simulink library "Lib_PFSys_CurrentLimiter_TMATS"  (R2017a)
settings: Solver=ode45  StartTime=0.0  StopTime=10.0  RelTol=1e-3  EnableMultiTasking=on
libraries: Lib_PF_BusLoadDC_TMATS x1
Description:
  | Thomas Modules
settings Model: Creator=jwchapm2  LastModifiedBy=glthoma1
settings DataIOCC: LimitDataPoints=on  SaveFormat=Array
settings OptimizationCC: ExpressionDepthLimit=2147483647  LifeSpan=inf
settings DebuggingCC: UnderspecifiedInitializationDetection=Classic  MergeDetectMultiDrivingBlocksExec=none  SolverPrmCheckMsg=warning  StateNameClashWarn=warning  SFUnexpectedBacktrackingDiag=warning  SFNoUnconditionalDefaultTransitionDiag=warning  SFExecutionAtInitializationDiag=none
settings HardwareCC: ProdBitPerPointer=32  ProdBitPerSizeT=32  ProdBitPerPtrDiffT=32  ProdLargestAtomicFloat=None  ProdIntDivRoundTo=Undefined  ProdEndianess=Unspecified  ProdWordSize=32  ProdHWDeviceType=32-bit Generic
settings ModelReferenceCC: PropagateSignalLabelsOutOfModel=off
settings GRTTargetCC: TargetLangStandard=C89/C90 (ANSI)  GeneratePreprocessorConditionals=Disable all
settings ConfigComp: CovMetricSettings=dw  CovHtmlReporting=on  CovSaveCumulativeToWorkspaceVar=on  CovSaveSingleToWorkspaceVar=on  CovExternalEMLEnable=off

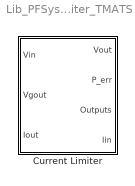
== system Lib_PFSys_CurrentLimiter_TMATS ==
  Current Limiter : Subsystem  mask(Current Limiter){ROn_M=0.01, ROff_M=0.01, IMax_M=1, IMin_M=-1, Rolloff_M=0}
      mask prompts: ROn_M "ROn_M - 'On' Resistance, Ohms"; ROff_M "ROff_M - 'Off' (HiZ) Resistance, Ohms"; IMax_M "IMax_M - Maximum Output Current, Amps"; IMin_M "IMin_M - Minimum Output Current, Amps"; Rolloff_M "Rolloff_M - Rolloff of Impedance Chracteristic as a function of Current (base of exponent)"
      mask help:
      | This block represents a generic current limiting device.
      | If the current through this device is within the upper/lower limits,
      | this device's impedance will be the "On Resistance." Otherwise
      | the impedance will be the "HiZ Resistance."
      |
      | If current is close to the bounds, the impedance will be
      | somewhere in between (the R vs I characteristic is sigmoidal.)
      | You can adjust the rolloff of the characteristic via the rolloff_M
      | parameter, which is the base of the sigmoid function's exponent.

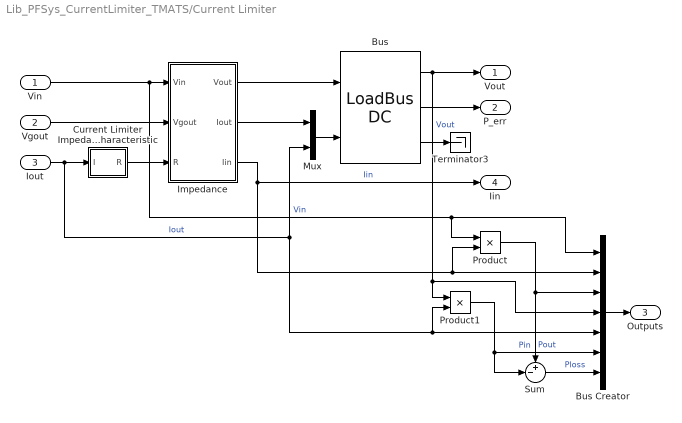
== system Lib_PFSys_CurrentLimiter_TMATS/Current Limiter ==
  Vin : Inport
  Vgout : Inport  Port=2
  Iout : Inport  Port=3
  Bus : Lib_PF_BusLoadDC_TMATS/LoadBus DC  PeInEN_M=off  P_M=0  BlkNm_M=double(gcb)
  Bus Creator : BusCreator  Inputs=7
  Current Limiter Impedance Characteristic : Subsystem
  Impedance : Subsystem
  Mux : Mux  Inputs=2
  Product : Product
  Product1 : Product
  Sum : Sum  Inputs=+-|
  Terminator3 : Terminator
  Vout : Outport
  P_err : Outport  Port=2
  Outputs : Outport  Port=3
  Iin : Outport  Port=4
  wires:
  Iout/1 -> Current Limiter Impedance Characteristic/1(I), Mux/2, Product1/2, Bus Creator/5  "Iout"
  Impedance/2(Iout) -> Mux/1
  Bus/1 -> Product1/1, Bus Creator/4, Vout/1  "Vout"
  Product1/1 -> Bus Creator/6, Sum/2  "Pout"
  Bus Creator/1 -> Outputs/1
  Vin/1 -> Product/1, Bus Creator/1, Impedance/1(Vin)  "Vin"
  Impedance/3(Iin) -> Product/2, Bus Creator/2, Iin/1  "Iin"
  Impedance/1(Vout) -> Bus/1
  Mux/1 -> Bus/2
  Vgout/1 -> Impedance/2(Vgout)
  Sum/1 -> Bus Creator/7  "Ploss"
  Bus/2 -> P_err/1
  Product/1 -> Bus Creator/3, Sum/1  "Pin"
  Bus/3 -> Terminator3/1
  Current Limiter Impedance Characteristic/1(R) -> Impedance/3(R)

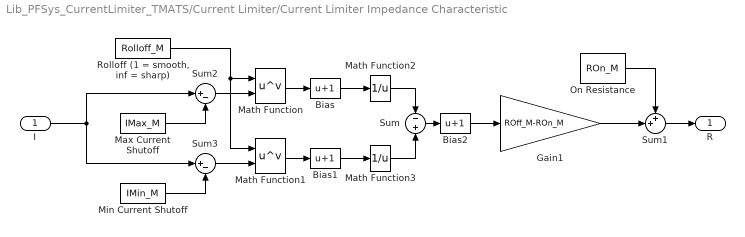
== system Lib_PFSys_CurrentLimiter_TMATS/Current Limiter/Current Limiter Impedance Characteristic ==
  I : Inport
  Bias : Bias  Bias=1
  Bias1 : Bias  Bias=1
  Bias2 : Bias  Bias=1
  Gain1 : Gain  Gain=ROff_M-ROn_M
  Math Function : Math  Operator=pow  SaturateOnIntegerOverflow=on
  Math Function1 : Math  Operator=pow  SaturateOnIntegerOverflow=on
  Math Function2 : Math  Operator=reciprocal  SaturateOnIntegerOverflow=on
  Math Function3 : Math  Operator=reciprocal  SaturateOnIntegerOverflow=on
  Max Current Shutoff : Constant  Value=IMax_M
  Min Current Shutoff : Constant  Value=IMin_M
  On Resistance : Constant  Value=ROn_M
  "Rolloff (1 = smooth, inf = sharp)" : Constant  Value=Rolloff_M
  Sum : Sum  Inputs=-+
  Sum1 : Sum  Inputs=++|
  Sum2 : Sum  Inputs=|+-
  Sum3 : Sum  Inputs=|+-
  R : Outport
  wires:
  Math Function3/1 -> Sum/2
  Bias/1 -> Math Function2/1
  Bias1/1 -> Math Function3/1
  Math Function1/1 -> Bias1/1
  Math Function2/1 -> Sum/1
  Math Function/1 -> Bias/1
  Sum3/1 -> Math Function1/2
  Sum2/1 -> Math Function/2
  I/1 -> Sum3/1, Sum2/1
  Min Current Shutoff/1 -> Sum3/2
  Max Current Shutoff/1 -> Sum2/2
  Gain1/1 -> Sum1/2
  On Resistance/1 -> Sum1/1
  Bias2/1 -> Gain1/1
  "Rolloff (1 = smooth, inf = sharp)"/1 -> Math Function/1, Math Function1/1
  Sum1/1 -> R/1
  Sum/1 -> Bias2/1

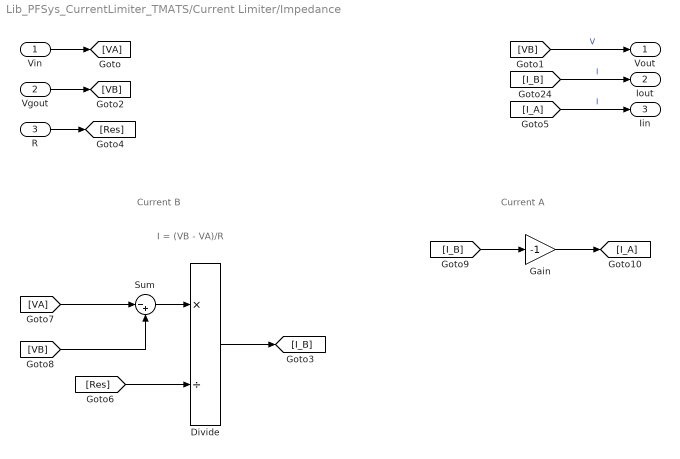
== system Lib_PFSys_CurrentLimiter_TMATS/Current Limiter/Impedance ==
  note: Current A
  note: Current B
  note: I = (VB - VA)/R
  Vin : Inport
  Vgout : Inport  Port=2
  R : Inport  Port=3
  Divide : Product  Inputs=*/
  Gain : Gain  Gain=-1
  Sum : Sum  Inputs=|-+
  Vout : Outport
  Iout : Outport  Port=2
  Iin : Outport  Port=3
  wires:
  Gain/1 -> [I_A]
  [I_B] -> Gain/1
  [Res] -> Divide/2
  Sum/1 -> Divide/1
  Divide/1 -> [I_B]
  [VA] -> Sum/1
  [VB] -> Sum/2
  [I_B] -> Iout/1  "I"
  R/1 -> [Res]
  [VB] -> Vout/1  "V"
  Vgout/1 -> [VB]
  [I_A] -> Iin/1  "I"
  Vin/1 -> [VA]
